simulink model "model_wahadla_2rzedu"  (R2024a)
settings: Solver=VariableStepAuto  StartTime=0.0  StopTime=10.0  RelTol=1e-3
InitFcn:
  | %%%%%PARAMETRY%%%%%
  | % m - masa
  | % J - moment bezwładności względem środka masy
  | % tau - moment obrotowy
  | % l - długość wahadła od punktu obrotu do środka masy
  | % b - ???
  | % mi - ???
  | m = 0.5;
  | J = 0.01;
  | tau = 1;
  | l = 0.5;
  | b = 0.02;
  | mi = 0.023;
  | g = 9.81;
settings Model: Creator=dyksi  LastModifiedBy=dyksi

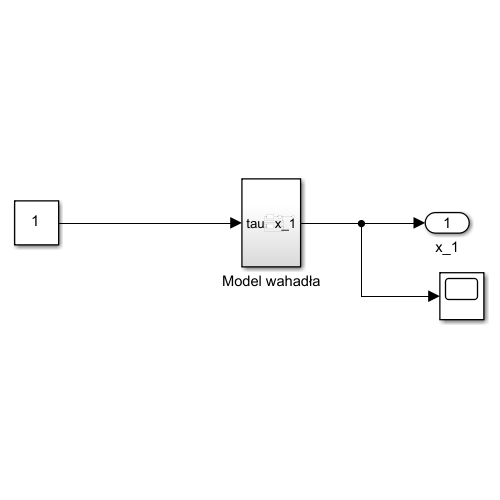
[thumbnail: Simulink's stored preview of the top-level diagram]
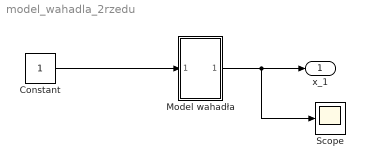
== system model_wahadla_2rzedu ==
  Constant : Constant
  Model wahadła : Subsystem
  Scope : Scope
  x_1 : Outport
  wires:
  Constant/1 -> Model wahadła/1(tau)
  Model wahadła/1(x_1) -> Scope/1, x_1/1

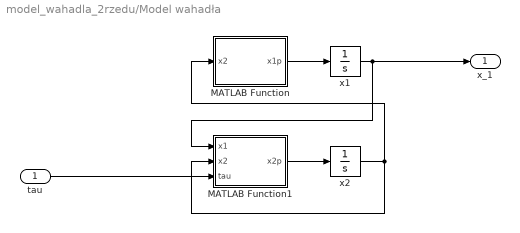
== system model_wahadla_2rzedu/Model wahadła ==
  tau : Inport
  MATLAB Function : MATLAB Function  TreatAsAtomicUnit=on
  MATLAB Function1 : MATLAB Function  TreatAsAtomicUnit=on
  x1 : Integrator
  x2 : Integrator
  x_1 : Outport
  wires:
  x2/1 -> MATLAB Function1/2(x2), MATLAB Function/1(x2)
  x1/1 -> x_1/1, MATLAB Function1/1(x1)
  MATLAB Function/1(x1p) -> x1/1
  tau/1 -> MATLAB Function1/3(tau)
  MATLAB Function1/1(x2p) -> x2/1

== matlab function model_wahadla_2rzedu/Model wahadła/MATLAB Function ==
  data: x2 input; x1p output
function x1p = fcn(x2)

x1p = x2;

== matlab function model_wahadla_2rzedu/Model wahadła/MATLAB Function1 ==
  data: x1 input; x2p output; x2 input; tau input
function x2p = fcn(x1,x2,tau)
m = 0.672;
l = 0.5;
g = 9.81;
J = 0.0021;
mi = 0.023;
b = 0.0051;
x2p = 1/(m*l^2+J) * (tau - b*x2 - mi*sign(x2) - l*m*g*cos(x1));
%
